simulink model "Washing_machine"  (R2024b)
settings: Solver=VariableStepAuto  StartTime=0.0  StopTime=inf  RelTol=1e-3
settings Model: PacingRate=5  Creator=rohan  LastModifiedBy=rohan

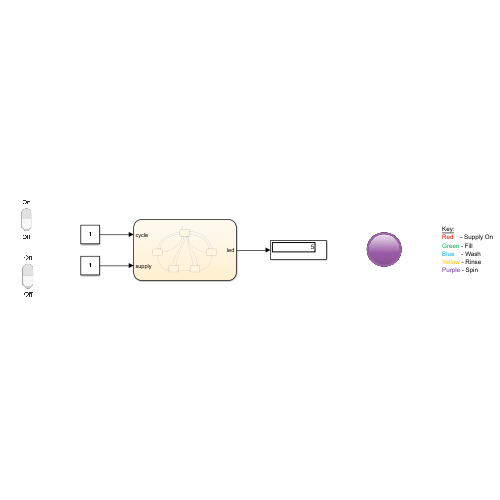
[thumbnail: Simulink's stored preview of the top-level diagram]
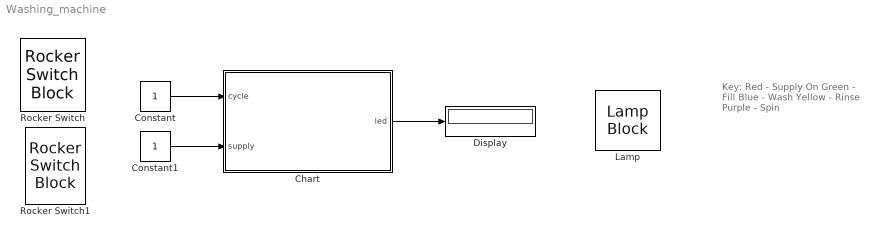
== system Washing_machine ==
  note: Key:
      | Red - Supply On
      | Green - Fill
      | Blue - Wash
      | Yellow - Rinse
      | Purple - Spin
  Chart : Stateflow chart  TreatAsAtomicUnit=on
  Constant : Constant
  Constant1 : Constant
  Display : Display
  Lamp : LampBlock  LabelPosition=Hide
  Rocker Switch : RockerSwitchBlock  LabelPosition=Hide
      settings: Values={{'Off', 'On'}, [0 1]}
  Rocker Switch1 : RockerSwitchBlock  LabelPosition=Hide
      settings: Values={{'Off', 'On'}, [0 1]}
  wires:
  Constant/1 -> Chart/1(cycle)
  Constant1/1 -> Chart/2(supply)
  Chart/1(led) -> Display/1

== stateflow chart Washing_machine/Chart ==
  state Idle
    entry:
    led=1
  state Fill
    led=2
  state Spin
    led=5
  state Wash
    led=3
  state Rinse
    led=4
  (default) -> Idle : {state=0}
  Spin -> Idle [order 1] : after(40,sec){state=0}
  Idle -> Fill [order 1] : [cycle==1 &&...
      | supply==1&&state==0]
  Idle -> Fill [order 5] : [cycle==1&&state==1]
  Idle -> Spin [order 2] : [cycle==1&&state==4]
  Fill -> Idle [order 2] : [cycle==0]
      | {state=1}
  Wash -> Idle [order 2] : [cycle==0]
  Idle -> Wash [order 4] : [cycle==1&& ...
      | state==2]
  Rinse -> Idle [order 2] : [cycle==0]
  Idle -> Rinse [order 3] : [cycle==1&&state==3]
  Spin -> Idle [order 2] : [cycle==0]
  Fill -> Wash [order 1] : after(30,sec){state=2}
  Rinse -> Spin [order 1] : after(40,sec){state=4}
  Wash -> Rinse [order 1] : after(40,sec){state=3}
  data: cycle input; supply input; led output; state local; s local
